simulink library "motohawk_engine_motoshare_lib"  (Simulink 6.3)
undefined symbols (not defined in the file or in its folder): cast_val, IndPowerMax, lookup_group, motohawk_tex, motohawk_vardec_config_group, motohawk_vardec_path, SampleTime, SteadyStateECT, txtTitle, WarmUpTimeConst
libraries: MotoHawk_lib x211, motohawk_control_primitives_lib x20, motohawk_annotations_lib x7, motohawk_engine_lib x5, AutoDoc_lib x4, motohawk_control_primitives_lib_new x3, motohawk_control_primitives_motoshare_lib x2
(part 6 of 7)

== system motohawk_engine_motoshare_lib/Linear Sensor Characterization w Adapt/Faults ==
  RawADC : Inport
  AdaptLimits : Inport  Port=2
  Bus Selector : BusSelector  OutputSignals=adapt_lo_min,adapt_hi_max
  Logical Operator : Logic  AllPortsSameDT=off  OutDataTypeMode=Boolean
  Logical Operator1 : Logic  AllPortsSameDT=off  OutDataTypeMode=Boolean
  Logical Operator2 : Logic  Operator=NOT  AllPortsSameDT=off  OutDataTypeMode=Boolean
  Logical Operator3 : Logic  Operator=NOT  AllPortsSameDT=off  OutDataTypeMode=Boolean
  Relational Operator1 : RelationalOperator  Operator=<
  Relational Operator3 : RelationalOperator  Operator=>
  Relational Operator4 : RelationalOperator  Operator=<
  Relational Operator5 : RelationalOperator  Operator=>
  motohawk_calibration5 : MotoHawk_lib/Calibration & Probing Blocks/motohawk_calibration  nam=[prefix 'RangeHiLimit']  val=1013  storage=Calibration  show_more=on  name_source=Use Parameter  data_type=Inherit from 'Default Value'  read_level=1  write_level=1  ovr_cals=on  view_as=Number  enum_struct={'Disabled', 'Enabled'}  vector_style=Wide Row  use_help_units=on  help='Hi limit of input signal which sets fault'  units='ADC'  use_header_enum=off  row_header_enum={}  col_header_enum={}  use_min_max=off  min_val=-inf  max_val=inf  use_precision=off  precision=''  gain=1  offset=0  exp=1  use_mototune_group=on  mototune_group=[group ' | ' nam ' Config']
  motohawk_calibration6 : MotoHawk_lib/Calibration & Probing Blocks/motohawk_calibration  nam=[prefix 'RangeLoLimit']  val=10  storage=Calibration  show_more=on  name_source=Use Parameter  data_type=Inherit from 'Default Value'  read_level=1  write_level=1  ovr_cals=on  view_as=Number  enum_struct={'Disabled', 'Enabled'}  vector_style=Wide Row  use_help_units=on  help='Low limit of input signal which sets fault'  units='ADC'  use_header_enum=off  row_header_enum={}  col_header_enum={}  use_min_max=off  min_val=-inf  max_val=inf  use_precision=off  precision=''  gain=1  offset=0  exp=1  use_mototune_group=on  mototune_group=[group ' | ' nam ' Config']
  motohawk_fault_def2 : MotoHawk_lib/Fault Management Blocks/motohawk_fault_def  nam=[prefix 'AdaptHi']  mode=Enabled  id=[]  x=25  y=50  input_suspected=on  indeterminate=off  increment_xy=on  downsample_count=1  ovr_cals=on  ovr_actions=on  show_actions=off  action1_name=''  action1_cond=(None)  action2_name=''  action2_cond=(None)  action3_name=''  action3_cond=(None)  action4_name=''  action4_cond=(None)
  motohawk_fault_def4 : MotoHawk_lib/Fault Management Blocks/motohawk_fault_def  nam=[prefix 'RangeHi']  mode=Enabled  id=[]  x=25  y=50  input_suspected=on  indeterminate=off  increment_xy=on  downsample_count=1  ovr_cals=on  ovr_actions=on  show_actions=off  action1_name=''  action1_cond=(None)  action2_name=''  action2_cond=(None)  action3_name=''  action3_cond=(None)  action4_name=''  action4_cond=(None)
  motohawk_fault_def5 : MotoHawk_lib/Fault Management Blocks/motohawk_fault_def  nam=[prefix 'RangeLo']  mode=Enabled  id=[]  x=25  y=50  input_suspected=on  indeterminate=off  increment_xy=on  downsample_count=1  ovr_cals=on  ovr_actions=on  show_actions=off  action1_name=''  action1_cond=(None)  action2_name=''  action2_cond=(None)  action3_name=''  action3_cond=(None)  action4_name=''  action4_cond=(None)
  motohawk_fault_def8 : MotoHawk_lib/Fault Management Blocks/motohawk_fault_def  nam=[prefix 'AdaptLo']  mode=Enabled  id=[]  x=25  y=50  input_suspected=on  indeterminate=off  increment_xy=on  downsample_count=1  ovr_cals=on  ovr_actions=on  show_actions=off  action1_name=''  action1_cond=(None)  action2_name=''  action2_cond=(None)  action3_name=''  action3_cond=(None)  action4_name=''  action4_cond=(None)
  wires:
  AdaptLimits/1 -> Bus Selector/1
  Bus Selector/1 -> Relational Operator1/2  "<adapt_lo_min>"
  Bus Selector/2 -> Relational Operator3/2  "<adapt_hi_max>"
  RawADC/1 -> Relational Operator4/1, Relational Operator5/1, Relational Operator1/1, Relational Operator3/1
  motohawk_calibration6/1 -> Relational Operator4/2
  motohawk_calibration5/1 -> Relational Operator5/2
  Relational Operator4/1 -> motohawk_fault_def5/1, Logical Operator2/1
  Relational Operator5/1 -> motohawk_fault_def4/1, Logical Operator3/1
  Logical Operator/1 -> motohawk_fault_def8/1
  Logical Operator1/1 -> motohawk_fault_def2/1
  Relational Operator1/1 -> Logical Operator/2
  Relational Operator3/1 -> Logical Operator1/2
  Logical Operator2/1 -> Logical Operator/1
  Logical Operator3/1 -> Logical Operator1/1

== system motohawk_engine_motoshare_lib/Load, Torque, Power, Work - Using APC/Calculate Power and Work ==
  IndTorque (N*m) : Inport
  RPM : Inport  Port=2
  Data Type Conversion : DataTypeConversion  SaturateOnIntegerOverflow=on  RndMeth=Zero
  Ground : Ground
  Integrate Power to Compute Work : motohawk_control_primitives_lib/Integrator  samp_time=SampleTime
  Mux1 : Mux  Inputs=2
  Torque to Power : Fcn  Expr=u(1)*u(2)*pi/30000
  motohawk_TitleBlock : motohawk_annotations_lib/motohawk_TitleBlock  BlockType_='Mototron_Title_Block'  ttl='Calculate Observed Engine States, such as Load, Torque, and Power\newline\rmUsing Airflow rate, calculate Air per Cylinder, and lookup Load and Torque values.'  copyright="'THE INFORMATION CONTAINED IN THIS\\newlineDRAWING IS THE SOLE PROPERTY OF\\newlineMOTOTRON.  ANY REPRODUCTION IN\\newline PART OR AS A WHOLE WITHOUT THE\\newlineWRITTEN PERMISSION OF MOTOTRON\\newline IS PROHIBITED.\\fontsize{16}\\rm\\copyright\\rm\\fontsize{10} 2005'"  address='\fontsize{22}\it\fontname{Arial Black}MotoTron Corporation \fontname{Arial}\fontsize{10}\newline505 Marion Road, Oshkosh, WI, 54901\newlinewww.mototron.com (734) 822-7700'  image_file='mh.jpg'  pretty_print=on  edit_text=[motohawk_tex(get_param(bdroot, 'Description')) '\rm\newline' motohawk_tex(get_param(gcs, 'Name'))]  edit_as=6
  motohawk_calibration : MotoHawk_lib/Calibration & Probing Blocks/motohawk_calibration  nam='IndWorkMax'  val=inf  storage=Calibration  show_more=on  name_source=Use Parameter  data_type=Inherit from 'Default Value'  read_level=1  write_level=1  ovr_cals=on  view_as=Number  enum_struct={'Disabled', 'Enabled'}  vector_style=Wide Row  use_help_units=on  help='Maximum Indicated Work'  units='kJ'  use_header_enum=off  row_header_enum={}  col_header_enum={}  use_min_max=off  min_val=-inf  max_val=inf  use_precision=off  precision=''  gain=1  offset=0  exp=1  use_mototune_group=on  mototune_group=lookup_group(gcb)
  motohawk_probe : MotoHawk_lib/Calibration & Probing Blocks/motohawk_probe  nam='IndPower'  show_more=on  name_source=Use Parameter  read_level=1  view_as=Number  enum_struct={'Disabled', 'Enabled'}  vector_style=Wide Row  use_help_units=on  help='Indicated Power'  units='kW'  use_header_enum=off  row_header_enum={}  col_header_enum={}  use_precision=off  precision=''  gain=1  offset=0  exp=1  use_mototune_group=on  mototune_group=lookup_group(gcb)
  motohawk_probe1 : MotoHawk_lib/Calibration & Probing Blocks/motohawk_probe  nam='IndWork'  show_more=on  name_source=Use Parameter  read_level=1  view_as=Number  enum_struct={'Disabled', 'Enabled'}  vector_style=Wide Row  use_help_units=on  help='Indicated Work'  units='kJ'  use_header_enum=off  row_header_enum={}  col_header_enum={}  use_precision=off  precision=''  gain=1  offset=0  exp=1  use_mototune_group=on  mototune_group=lookup_group(gcb)
  IndPower (kW) : Outport
  IndWork (kJ) : Outport  Port=2
  wires:
  Mux1/1 -> Data Type Conversion/1
  Data Type Conversion/1 -> Torque to Power/1
  Torque to Power/1 -> Integrate Power to Compute Work/1, IndPower (kW)/1, motohawk_probe/1
  Integrate Power to Compute Work/1 -> IndWork (kJ)/1, motohawk_probe1/1
  motohawk_calibration/1 -> Integrate Power to Compute Work/5
  IndTorque (N*m)/1 -> Mux1/1
  RPM/1 -> Mux1/2
  Ground/1 -> Integrate Power to Compute Work/3, Integrate Power to Compute Work/2, Integrate Power to Compute Work/4

== system motohawk_engine_motoshare_lib/Mass Flow to Charge Mass Transform/Multiply and Divide, avoiding divde by zero ==
  X1 : Inport
  "X2 " : Inport  Port=2
  Divide1 : Inport  Port=3
  Divide2 : Inport  Port=4
  Enable : EnablePort  StatesWhenEnabling=reset
  charge mass : Product  Inputs=**//  SaturateOnIntegerOverflow=on  InputSameDT=on
  " " : Outport
  wires:
  charge mass/1 -> " "/1
  "X2 "/1 -> charge mass/2
  X1/1 -> charge mass/1
  Divide1/1 -> charge mass/3
  Divide2/1 -> charge mass/4

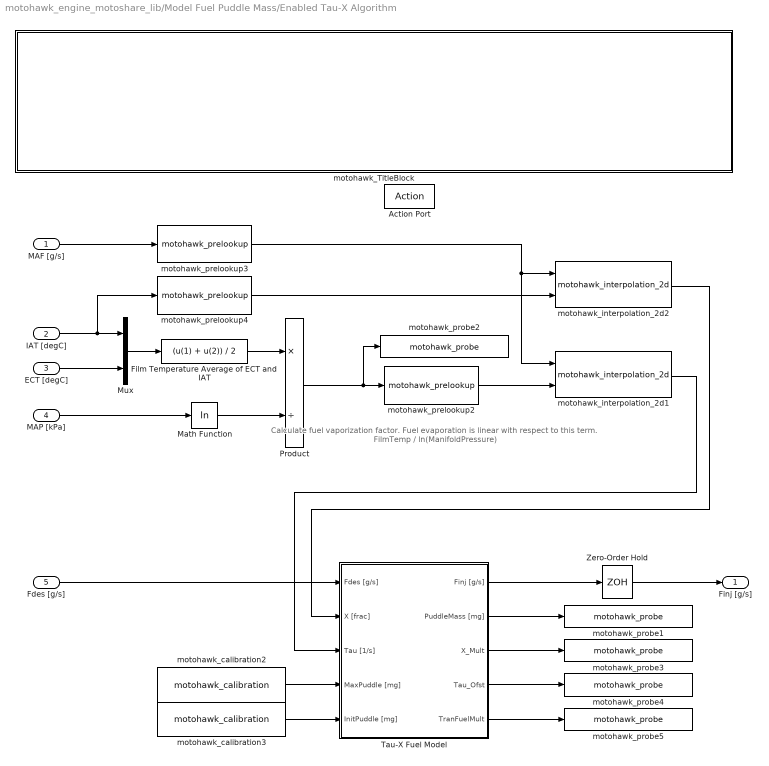
== system motohawk_engine_motoshare_lib/Model Fuel Puddle Mass/Enabled Tau-X Algorithm ==
  note: Calculate fuel vaporization factor.
      | Fuel evaporation is linear with respect to this term.
      | FilmTemp / ln(ManifoldPressure)
  MAF [g/s] : Inport
  IAT [degC] : Inport  Port=2
  ECT [degC] : Inport  Port=3
  MAP [kPa] : Inport  Port=4
  Fdes [g/s] : Inport  Port=5
  Action Port : ActionPort  InitializeStates=reset
  Film Temperature Average of ECT and IAT : Fcn  Expr=(u(1) + u(2)) / 2
  Math Function : Math  Operator=log  SaturateOnIntegerOverflow=on
  Mux : Mux  Inputs=2
  Product : Product  Inputs=*/  SaturateOnIntegerOverflow=on  InputSameDT=on
  Tau-X Fuel Model : Subsystem  mask{samp_time=SampleTime}
      mask prompts: samp_time "Sample Time"
      mask Display:
      | patch([0 0 1 1], 0.5*[0 0.075 0.075 0], [230/255 0/255 0/255])
      | patch([0 0 1 1], 0.5*[0.025 0.05 0.05 0.025], [150/255 0/255 0/255])
      | patch([0 0 1 1], 0.5*[0 0.025 0.025 0], [0/255 0/255 0/255])
      | 
      | disp('TRANSIENT FUELING\nTAU-X MODEL');
  Zero-Order Hold : ZeroOrderHold  SampleTime=-1
  motohawk_TitleBlock : Subsystem  mask{BlockType_='Mototron_Title_Block', ttl=[txtTitle '\newline\rmPer-Cylinder Transient Fueling Model\newlineSchedule Tau and X parameters on RPM and load'], im=mh.jpg}
      mask prompts: ttl "Description"; im "Image FIle"
      mask init:
      | set_param(gcb,'BlockType_','''Mototron_Title_Block''')
      | set_param(gcb,'MaskVisibilityString','off,on,on');
      mask Display:
      | image(imread(im),[0.31 0.66 0.31 0.35])
      | 
      | plot([0 0 1 1 0],[0 1 1 0 0])
      | plot([.3 1],[0.65 0.65])
      | plot([.3 .3],[0.1 1.0])
      | plot([0 1],[0.1 0.1])
      | plot([0.91 0.91],[0 0.1])
      | text(1,1,'\fontsize{22}\it\fontname{Arial Black}MotoTron Corporation \fontname{Arial}\fontsize{10}\newline505 Marion Road, Oshkosh, WI, 54901\newlinewww.mototron.com (734) 822-7700','verticalAlignment','Top','horizontalAlignment','Right','texmode','on')
      | text(0.01,1,['\fontsize{14}\it\bfPROPRIETARY\newlineAND CONFIDENTIAL\newline\fontsize{10}
      | THE INFORMATION CONTAINED IN THIS\newline
      | DRAWING IS THE SOLE PROPERTY OF\newline
      | MOTOTRON.  ANY REPRODUCTION IN\newline
      | PART OR AS A WHOLE WITHOUT THE\newline
      | WRITTEN PERMISSION OF MOTOTRON\newline
      | IS PROHIBITED.\fontsize{16}\rm\copyright\rm\fontsize{10} 2004' ],'verticalAlignment','Top','horizontalAlignment','Left','texmode','on')
      | 
      | text(0.9,0,['\fontsize{11}\bfPath: \rm' strrep(motohawk_vardec_path(gcb),'_','\_')],'verticalAlignment','Bottom','horizontalAlignment','Right','texmode','on')
      | text(0.31,0.65,['\fontsize{10}\bfDescription:'],'verticalAlignment','Top','horizontalAlignment','Left','texmode','on')
      | 
      | text(0.31,0.55,['\fontsize{14}\bf' ttl],'verticalAlignment','Top','horizontalAlignment','Left','texmode','on')
      | text(0.99,0,['\fontsize{11}\bfREV: \rm' motohawk_build_version],'verticalAlignment','Bottom','horizontalAlignment','Right','texmode','on')
  motohawk_calibration2 : MotoHawk_lib/Calibration & Probing Blocks/motohawk_calibration  nam='TransientFuelMaxPuddle'  val=0  storage=Calibration  show_more=on  name_source=Use Parameter  data_type=Inherit from 'Default Value'  read_level=1  write_level=1  ovr_cals=on  view_as=Number  enum_struct={'Disabled', 'Enabled'}  vector_style=Wide Row  use_help_units=on  help='Maximum fuel puddle size'  units='mg'  use_header_enum=off  row_header_enum={}  col_header_enum={}  use_min_max=on  min_val=0  max_val=inf  use_precision=off  precision=''  gain=1  offset=0  exp=1  use_mototune_group=on  mototune_group=group_cal
  motohawk_calibration3 : MotoHawk_lib/Calibration & Probing Blocks/motohawk_calibration  nam='TransientFuelInitPuddle'  val=0  storage=Calibration  show_more=on  name_source=Use Parameter  data_type=Inherit from 'Default Value'  read_level=1  write_level=1  ovr_cals=on  view_as=Number  enum_struct={'Disabled', 'Enabled'}  vector_style=Wide Row  use_help_units=on  help='Initial fuel puddle size'  units='mg'  use_header_enum=off  row_header_enum={}  col_header_enum={}  use_min_max=on  min_val=0  max_val=inf  use_precision=off  precision=''  gain=1  offset=0  exp=1  use_mototune_group=on  mototune_group=group_cal
  motohawk_interpolation_2d1 : MotoHawk_lib/Lookup Tables/motohawk_interpolation_2d  nam='TransientFuelTau'  table_data=ones(5,5)  show_more=on  data_type=Inherit from 'Table Data'  storage=NonAdaptive  read_level=1  write_level=1  ovr_cals=on  use_help=on  help='Fuel evaporation time constant'  units='sec'  use_min_max=on  min_val=SampleTime  max_val=inf  use_precision=off  precision=''  gain=1  offset=0  exp=1  use_links=off  row_prelookup_block=''  col_prelookup_block=''  output_name=''  use_mototune_group=on  mototune_group=group_cal
  motohawk_interpolation_2d2 : MotoHawk_lib/Lookup Tables/motohawk_interpolation_2d  nam='TransientFuelX'  table_data=ones(5,5)  show_more=on  data_type=Inherit from 'Table Data'  storage=NonAdaptive  read_level=1  write_level=1  ovr_cals=on  use_help=on  help='Fraction of injected fuel to enter the puddle'  units='frac'  use_min_max=on  min_val=0  max_val=1  use_precision=off  precision=''  gain=1  offset=0  exp=1  use_links=off  row_prelookup_block=''  col_prelookup_block=''  output_name=''  use_mototune_group=on  mototune_group=group_cal
  motohawk_prelookup2 : MotoHawk_lib/Lookup Tables/motohawk_prelookup  nam='FuelVapFactor'  breakpoint_data=ones(1,5)  show_more=on  data_type=Inherit from 'Table Data'  storage=Constant  read_level=1  write_level=1  ovr_cals=on  use_help=on  help='Breakpoints for fuel vaporization factor'  units='degC/log(kPa)'  use_min_max=off  min_val=-inf  max_val=inf  use_precision=off  precision=''  gain=1  offset=0  exp=1  use_links=on  input_name=''  use_mototune_group=on  mototune_group='Indexes'
  motohawk_prelookup3 : MotoHawk_lib/Lookup Tables/motohawk_prelookup  nam='MAF05'  breakpoint_data=ones(1,5)  show_more=on  data_type=Inherit from 'Table Data'  storage=Constant  read_level=1  write_level=1  ovr_cals=on  use_help=on  help='Breakpoints for Mass Airflow'  units='g/s'  use_min_max=off  min_val=-inf  max_val=inf  use_precision=off  precision=''  gain=1  offset=0  exp=1  use_links=on  input_name='MAF'  use_mototune_group=on  mototune_group='Indexes'
  motohawk_prelookup4 : MotoHawk_lib/Lookup Tables/motohawk_prelookup  nam='IAT05'  breakpoint_data=ones(1,5)  show_more=on  data_type=Inherit from 'Table Data'  storage=Constant  read_level=1  write_level=1  ovr_cals=on  use_help=on  help='Breakpoints for intake air temperature'  units='degC'  use_min_max=off  min_val=-inf  max_val=inf  use_precision=off  precision=''  gain=1  offset=0  exp=1  use_links=on  input_name='IAT'  use_mototune_group=on  mototune_group='Indexes'
  motohawk_probe1 : MotoHawk_lib/Calibration & Probing Blocks/motohawk_probe  nam='TransientFuelPuddleMass'  show_more=on  name_source=Use Parameter  read_level=1  view_as=Number  enum_struct={'Disabled', 'Enabled'}  vector_style=Wide Row  use_help_units=on  help='Current modeled fuel puddle mass for Tau-X transient fuel'  units='mg'  use_header_enum=off  row_header_enum={}  col_header_enum={}  use_precision=off  precision=''  gain=1  offset=0  exp=1  use_mototune_group=on  mototune_group=group_dis
  motohawk_probe2 : MotoHawk_lib/Calibration & Probing Blocks/motohawk_probe  nam='FuelVapFactor'  show_more=on  name_source=Use Parameter  read_level=1  view_as=Number  enum_struct={'Disabled', 'Enabled'}  vector_style=Wide Row  use_help_units=on  help='Fuel vaporization factor - Fuel evaporation is linear with respect to this term'  units='degC/log(kPa)'  use_header_enum=off  row_header_enum={}  col_header_enum={}  use_precision=off  precision=''  gain=1  offset=0  exp=1  use_mototune_group=on  mototune_group=group_dis
  motohawk_probe3 : MotoHawk_lib/Calibration & Probing Blocks/motohawk_probe  nam='TransientFuel_X_Mult'  show_more=on  name_source=Use Parameter  read_level=1  view_as=Number  enum_struct={'Disabled', 'Enabled'}  vector_style=Wide Row  use_help_units=on  help='Multiplier on desired fuel flow due to X contribution (1/(1-X)).'  units=''  use_header_enum=off  row_header_enum={}  col_header_enum={}  use_precision=off  precision=''  gain=1  offset=0  exp=1  use_mototune_group=on  mototune_group=group_dis
  motohawk_probe4 : MotoHawk_lib/Calibration & Probing Blocks/motohawk_probe  nam='TransientFuel_Tau_Ofst'  show_more=on  name_source=Use Parameter  read_level=1  view_as=Number  enum_struct={'Disabled', 'Enabled'}  vector_style=Wide Row  use_help_units=on  help='Offset applied to desired fuel flow based on Tau contribution (-M_pud/Tau).'  units='g/s'  use_header_enum=off  row_header_enum={}  col_header_enum={}  use_precision=off  precision=''  gain=1  offset=0  exp=1  use_mototune_group=on  mototune_group=group_dis
  motohawk_probe5 : MotoHawk_lib/Calibration & Probing Blocks/motohawk_probe  nam='TransientFuel_Total_Mult'  show_more=on  name_source=Use Parameter  read_level=1  view_as=Number  enum_struct={'Disabled', 'Enabled'}  vector_style=Wide Row  use_help_units=on  help='Total transient fuel multiplier applied to desired fuel flow resulting from Tau-X model.'  units=''  use_header_enum=off  row_header_enum={}  col_header_enum={}  use_precision=off  precision=''  gain=1  offset=0  exp=1  use_mototune_group=on  mototune_group=group_dis
  Finj [g/s] : Outport
  wires:
  Tau-X Fuel Model/5(TranFuelMult) -> motohawk_probe5/1
  Tau-X Fuel Model/4(Tau_Ofst) -> motohawk_probe4/1
  Tau-X Fuel Model/3(X_Mult) -> motohawk_probe3/1
  motohawk_calibration2/1 -> Tau-X Fuel Model/4(MaxPuddle [mg])
  motohawk_calibration3/1 -> Tau-X Fuel Model/5(InitPuddle [mg])
  Tau-X Fuel Model/2(PuddleMass [mg]) -> motohawk_probe1/1
  Mux/1 -> Film Temperature Average of ECT and IAT/1
  Film Temperature Average of ECT and IAT/1 -> Product/1
  Math Function/1 -> Product/2
  Product/1 -> motohawk_prelookup2/1, motohawk_probe2/1
  IAT [degC]/1 -> Mux/1, motohawk_prelookup4/1
  motohawk_prelookup3/1 -> motohawk_interpolation_2d2/1, motohawk_interpolation_2d1/1
  motohawk_prelookup4/1 -> motohawk_interpolation_2d2/2
  Fdes [g/s]/1 -> Tau-X Fuel Model/1(Fdes [g/s])
  MAF [g/s]/1 -> motohawk_prelookup3/1
  ECT [degC]/1 -> Mux/2
  MAP [kPa]/1 -> Math Function/1
  Tau-X Fuel Model/1(Finj [g/s]) -> Zero-Order Hold/1
  Zero-Order Hold/1 -> Finj [g/s]/1
  motohawk_prelookup2/1 -> motohawk_interpolation_2d1/2
  motohawk_interpolation_2d1/1 -> Tau-X Fuel Model/3(Tau [1/s])
  motohawk_interpolation_2d2/1 -> Tau-X Fuel Model/2(X [frac])

== system motohawk_engine_motoshare_lib/Model Fuel Puddle Mass/Pass-Through ==
  note: Simply pass-through desired fuel as injected fuel
      | when transient fueling is disabled
  Fdes [g/s] : Inport
  Action Port : ActionPort  InitializeStates=reset
  Finj [g/s] : Outport
  wires:
  Fdes [g/s]/1 -> Finj [g/s]/1

== system motohawk_engine_motoshare_lib/Model Fuel Puddle Mass/motohawk_TitleBlock ==

== system motohawk_engine_motoshare_lib/Non-Linear Sensor Characterization (eqn)/If Action Subsystem ==
  In : Inport
  Action Port : ActionPort
  Out : Outport
  wires:
  In/1 -> Out/1

== system motohawk_engine_motoshare_lib/Non-Linear Sensor Characterization (eqn)/If Action Subsystem2 ==
  In : Inport
  Action Port : ActionPort
  Out : Outport
  wires:
  In/1 -> Out/1

== system motohawk_engine_motoshare_lib/Non-Linear Sensor Characterization (tbl)/If Action Subsystem ==
  In : Inport
  Action Port : ActionPort
  Out : Outport
  wires:
  In/1 -> Out/1

== system motohawk_engine_motoshare_lib/Non-Linear Sensor Characterization (tbl)/If Action Subsystem1 ==
  In : Inport
  Action Port : ActionPort
  Out : Outport
  wires:
  In/1 -> Out/1

== system motohawk_engine_motoshare_lib/Non-Linear Sensor Characterization (tbl)/If Action Subsystem2 ==
  In : Inport
  Action Port : ActionPort
  Out : Outport
  wires:
  In/1 -> Out/1

== system motohawk_engine_motoshare_lib/Normalized Effective Combustion Chamber Temperature/CompareTo ==
  note: Check how input compares to 'val'
  In : Inport
  Constant : Constant  Value=val
  RelOp : RelationalOperator  Operator===  ZeroCross=off  InputSameDT=on
  Out : Outport
  wires:
  In/1 -> RelOp/1
  RelOp/1 -> Out/1
  Constant/1 -> RelOp/2

== system motohawk_engine_motoshare_lib/Normalized Effective Combustion Chamber Temperature/Integrate an offset to ECT  Reset offset when engine is stopped. ==
  Integrand : Inport
  Reset : Inport  Port=2
  Enable : EnablePort
  Constant : Constant  Value=0
  Constant1 : Constant  Value=0
  Constant2 : Constant  Value=inf
  Integrator : Subsystem  mask(Discrete Integrator){samp_time=SampleTime}
      mask prompts: samp_time "Sample Time"
      mask help:
      | Resetable integrator with upper and lower windup limits.
      |
      | If 'Sample Time' is -1, then extra code and RAM will be generated to dynamically calculate dt.
      mask Display:
      | patch([0 0 1 1], 0.75*[0 0.075 0.075 0], [230/255 0/255 0/255])
      | patch([0 0 1 1], 0.75*[0.025 0.05 0.05 0.025], [150/255 0/255 0/255])
      | patch([0 0 1 1], 0.75*[0 0.025 0.025 0], [0/255 0/255 0/255])
      | 
      | disp('\fontsize{16}\bf\it\int dt', 'texmode', 'on')
  ECT Offset : Outport
  wires:
  Constant/1 -> Integrator/4(Min)
  Constant1/1 -> Integrator/3(IC)
  Integrand/1 -> Integrator/1(In)
  Integrator/1(Out) -> ECT Offset/1
  Reset/1 -> Integrator/2(Rst)
  Constant2/1 -> Integrator/5(Max)

== system motohawk_engine_motoshare_lib/Normalized Effective Combustion Chamber Temperature/motohawk_TitleBlock ==

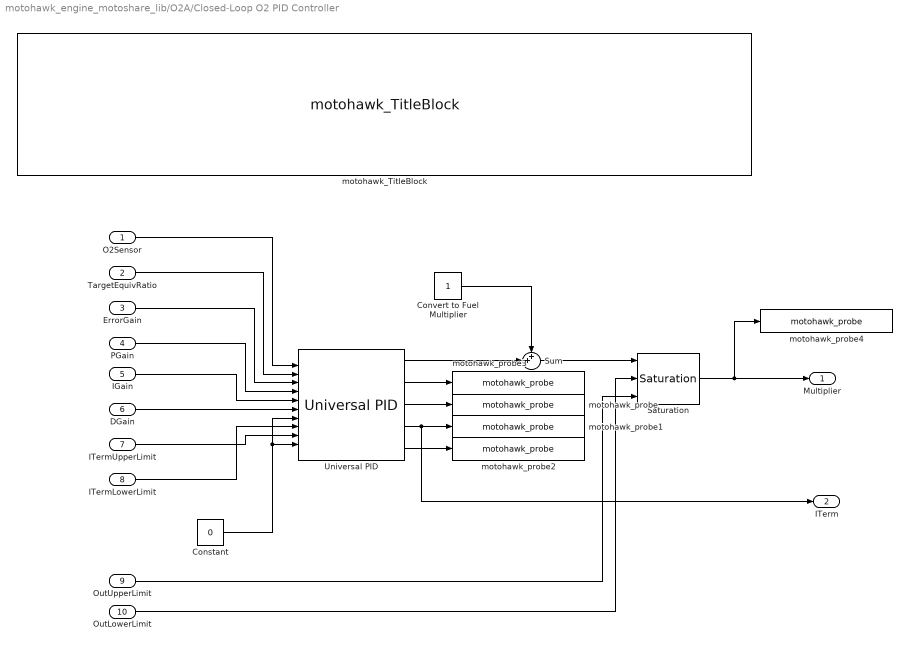
== system motohawk_engine_motoshare_lib/O2A/Closed-Loop O2 PID Controller ==
  O2Sensor : Inport
  TargetEquivRatio : Inport  Port=2
  ErrorGain : Inport  Port=3
  PGain : Inport  Port=4
  IGain : Inport  Port=5
  DGain : Inport  Port=6
  ITermUpperLimit : Inport  Port=7
  ITermLowerLimit : Inport  Port=8
  OutUpperLimit : Inport  Port=9
  OutLowerLimit : Inport  Port=10
  Constant : Constant  Value=0
  Convert to Fuel Multiplier : Constant
  Saturation : motohawk_control_primitives_lib/Saturation
  Sum : Sum  Inputs=++|  SaturateOnIntegerOverflow=on  InputSameDT=on
  Universal PID : motohawk_control_primitives_lib/Universal PID  Description=|  samp_time=-1
      | /* Name: ErrorGain Unit:mult ClassID:VAR StorageID:FLASH Access:RW4+RW3+NA2+NA1 TypeID:UINT4                   
      |    Gain:0.000000001 Min:0.000000000 Max:4.000000000 Format:10.9 UpdateID:REMOTE Help:"This gain is applied to "
      |    "the error term before it is used to calculate the P, I and D terms." VardecSig:6C */                       
      |                                                                                                                
      | /* Name: ITermLowerLim Unit:0 ClassID:VAR StorageID:FLASH Access:RW4+RW3+NA2+NA1 TypeID:SINT2 Gain:0.1         
      |    Min:-3276.8 Max:3276.7 Format:5.1 UpdateID:REMOTE Help:"Lower limit on the I-term value." VardecSig:6C */   
      |                                                                                                                
      | /* Name: ITermUpperLim ClassID:VAR StorageID:FLASH Access:RW4+RW3+NA2+NA1 TypeID:SINT2 Gain:0.1 Min:-3276.8    
      |    Max:3276.7 Format:5.1 UpdateID:REMOTE Help:"Upper limit on I-term value." VardecSig:6C */                   
      |                                                                                                                
      | /* Name: PIDOutLowerLim ClassID:VAR StorageID:FLASH Access:RW4+RW3+NA2+NA1 TypeID:SINT2 Gain:0.1               
      |    Min:-3276.8 Max:3276.7 Format:5.1 UpdateID:REMOTE Help:"Lower limit on PID output." VardecSig:6C */         
      |                                                                                                                
      | /* Name: PIDOutUpperLim ClassID:VAR StorageID:FLASH Access:RW4+RW3+NA2+NA1 TypeID:SINT2 Gain:0.1               
      |    Min:-3276.8 Max:3276.7 Format:3.1 UpdateID:REMOTE Help:"Upper limit on PID output." VardecSig:6C */
  motohawk_TitleBlock : motohawk_annotations_lib/motohawk_TitleBlock  BlockType_='Mototron_Title_Block'  ttl=[txtTitle '\newline\rmClosed-loop O2 Control - PID for Bank A']  copyright="'THE INFORMATION CONTAINED IN THIS\\newlineDRAWING IS THE SOLE PROPERTY OF\\newlineMOTOTRON.  ANY REPRODUCTION IN\\newline PART OR AS A WHOLE WITHOUT THE\\newlineWRITTEN PERMISSION OF MOTOTRON\\newline IS PROHIBITED.\\fontsize{16}\\rm\\copyright\\rm\\fontsize{10} 2005'"  address='\fontsize{22}\it\fontname{Arial Black}MotoTron Corporation \fontname{Arial}\fontsize{10}\newline505 Marion Road, Oshkosh, WI, 54901\newlinewww.mototron.com (734) 822-7700'  image_file='mh.jpg'  pretty_print=on  edit_text=[motohawk_tex(get_param(bdroot, 'Description')) '\rm\newline' motohawk_tex(get_param(gcs, 'Name'))]  edit_as=6
  motohawk_probe : MotoHawk_lib/Calibration & Probing Blocks/motohawk_probe  nam=['O2Control_PTerm' bank]  show_more=on  name_source=Use Parameter  read_level=1  view_as=Number  enum_struct={'Disabled', 'Enabled'}  vector_style=Wide Row  use_help_units=on  help=['Closed-loop O2 control P-Term, for bank ' bank]  units='mult'  use_header_enum=off  row_header_enum={}  col_header_enum={}  use_precision=off  precision=''  gain=1  offset=0  exp=1  use_mototune_group=on  mototune_group=display_group
  motohawk_probe1 : MotoHawk_lib/Calibration & Probing Blocks/motohawk_probe  nam=['O2Control_ITerm' bank]  show_more=on  name_source=Use Parameter  read_level=1  view_as=Number  enum_struct={'Disabled', 'Enabled'}  vector_style=Wide Row  use_help_units=on  help=['Closed-loop O2 control I-Term, for bank ' bank]  units='mult'  use_header_enum=off  row_header_enum={}  col_header_enum={}  use_precision=off  precision=''  gain=1  offset=0  exp=1  use_mototune_group=on  mototune_group=display_group
  motohawk_probe2 : MotoHawk_lib/Calibration & Probing Blocks/motohawk_probe  nam=['O2Control_DTerm' bank]  show_more=on  name_source=Use Parameter  read_level=1  view_as=Number  enum_struct={'Disabled', 'Enabled'}  vector_style=Wide Row  use_help_units=on  help=['Closed-loop O2 control D-Term, for bank ' bank]  units='mult'  use_header_enum=off  row_header_enum={}  col_header_enum={}  use_precision=off  precision=''  gain=1  offset=0  exp=1  use_mototune_group=on  mototune_group=display_group
  motohawk_probe3 : MotoHawk_lib/Calibration & Probing Blocks/motohawk_probe  nam=['O2Control_ErrorTerm' bank]  show_more=on  name_source=Use Parameter  read_level=1  view_as=Number  enum_struct={'Disabled', 'Enabled'}  vector_style=Wide Row  use_help_units=on  help=['Closed-loop O2 control error-term, for bank ' bank]  units='mult'  use_header_enum=off  row_header_enum={}  col_header_enum={}  use_precision=off  precision=''  gain=1  offset=0  exp=1  use_mototune_group=on  mototune_group=display_group
  motohawk_probe4 : MotoHawk_lib/Calibration & Probing Blocks/motohawk_probe  nam=['O2FuelMult' bank]  show_more=on  name_source=Use Parameter  read_level=1  view_as=Number  enum_struct={'Disabled', 'Enabled'}  vector_style=Wide Row  use_help_units=on  help=['Closed-loop O2 control fuel multiplier, for bank ' bank]  units='mult'  use_header_enum=off  row_header_enum={}  col_header_enum={}  use_precision=off  precision=''  gain=1  offset=0  exp=1  use_mototune_group=on  mototune_group=display_group
  Multiplier : Outport
  ITerm : Outport  Port=2
  wires:
  Universal PID/2 -> motohawk_probe3/1
  OutLowerLimit/1 -> Saturation/2
  ITermLowerLimit/1 -> Universal PID/8
  ITermUpperLimit/1 -> Universal PID/9
  Sum/1 -> Saturation/1
  Universal PID/1 -> Sum/2
  Convert to Fuel Multiplier/1 -> Sum/1
  OutUpperLimit/1 -> Saturation/3
  DGain/1 -> Universal PID/6
  IGain/1 -> Universal PID/5
  PGain/1 -> Universal PID/4
  ErrorGain/1 -> Universal PID/3
  TargetEquivRatio/1 -> Universal PID/2
  O2Sensor/1 -> Universal PID/1
  Saturation/1 -> motohawk_probe4/1, Multiplier/1
  Universal PID/5 -> motohawk_probe2/1
  Constant/1 -> Universal PID/7, Universal PID/10
  Universal PID/4 -> ITerm/1, motohawk_probe1/1
  Universal PID/3 -> motohawk_probe/1

== system motohawk_engine_motoshare_lib/O2A/Equivalence Ratio Perturbation ==
  note: When low, switch to rich.
      | When high, switch to lean.
  O2Sensor : Inport
  DesEquivRatio : Inport  Port=2
  RichEquivRatioTargetDelta : Inport  Port=3
  LeanEquivRatioTargetDelta : Inport  Port=4
  RichEquivRatioSwPtDelta : Inport  Port=5
  LeanEquivRatioSwPtDelta : Inport  Port=6
  Hysteresis : Subsystem
  LT : RelationalOperator  ZeroCross=off  InputSameDT=on
  LT1 : RelationalOperator  Operator=<=  ZeroCross=off  InputSameDT=on
  Logical Operator : Logic  Operator=NOT
  Sum1 : Sum  SaturateOnIntegerOverflow=on
  Sum2 : Sum  Inputs=-+  SaturateOnIntegerOverflow=on
  Sum3 : Sum  SaturateOnIntegerOverflow=on
  Sum4 : Sum  Inputs=+-  SaturateOnIntegerOverflow=on
  Switch2 : Switch  Threshold=1  ZeroCross=off  InputSameDT=on
  motohawk_TitleBlock : motohawk_annotations_lib/motohawk_TitleBlock  BlockType_='Mototron_Title_Block'  ttl=[txtTitle '\newline\rmO2 Control Target Equivalence Ratio Perturbation around Stoichiometric']  copyright="'THE INFORMATION CONTAINED IN THIS\\newlineDRAWING IS THE SOLE PROPERTY OF\\newlineMOTOTRON.  ANY REPRODUCTION IN\\newline PART OR AS A WHOLE WITHOUT THE\\newlineWRITTEN PERMISSION OF MOTOTRON\\newline IS PROHIBITED.\\fontsize{16}\\rm\\copyright\\rm\\fontsize{10} 2005'"  address='\fontsize{22}\it\fontname{Arial Black}MotoTron Corporation \fontname{Arial}\fontsize{10}\newline505 Marion Road, Oshkosh, WI, 54901\newlinewww.mototron.com (734) 822-7700'  image_file='mh.jpg'  pretty_print=on  edit_text=[motohawk_tex(get_param(bdroot, 'Description')) '\rm\newline' motohawk_tex(get_param(gcs, 'Name'))]  edit_as=6
  motohawk_fault_def : MotoHawk_lib/Fault Management Blocks/motohawk_fault_def  nam=['O2FailedLean',bank]  mode=Enabled  id=[]  x=25  y=50  input_suspected=on  indeterminate=off  increment_xy=on  downsample_count=1  ovr_cals=on  ovr_actions=on  show_actions=off  action1_name=''  action1_cond=(None)  action2_name=''  action2_cond=(None)  action3_name=''  action3_cond=(None)  action4_name=''  action4_cond=(None)
  motohawk_fault_def1 : MotoHawk_lib/Fault Management Blocks/motohawk_fault_def  nam=['O2FailedRich',bank]  mode=Enabled  id=[]  x=25  y=50  input_suspected=on  indeterminate=off  increment_xy=on  downsample_count=1  ovr_cals=on  ovr_actions=on  show_actions=off  action1_name=''  action1_cond=(None)  action2_name=''  action2_cond=(None)  action3_name=''  action3_cond=(None)  action4_name=''  action4_cond=(None)
  Target Phi : Outport
  wires:
  Logical Operator/1 -> Switch2/2
  O2Sensor/1 -> LT/1, LT1/1
  Hysteresis/1("Out (Lo=0, Hi=1)") -> Logical Operator/1
  LT1/1 -> motohawk_fault_def/1, Hysteresis/2(Lo)  "BelowLean"
  LT/1 -> motohawk_fault_def1/1, Hysteresis/1(Hi)  "AboveRich"
  RichEquivRatioTargetDelta/1 -> Sum1/1
  LeanEquivRatioTargetDelta/1 -> Sum2/1
  Sum1/1 -> Switch2/1
  Sum2/1 -> Switch2/3
  LeanEquivRatioSwPtDelta/1 -> Sum4/2
  RichEquivRatioSwPtDelta/1 -> Sum3/2
  DesEquivRatio/1 -> Sum3/1, Sum4/1, Sum2/2, Sum1/2
  Switch2/1 -> Target Phi/1
  Sum4/1 -> LT1/2
  Sum3/1 -> LT/2

== system motohawk_engine_motoshare_lib/O2A/O2 Calibrations ==
  Bus Creator : BusCreator  Inputs=12
  motohawk_TitleBlock : motohawk_annotations_lib/motohawk_TitleBlock  BlockType_='Mototron_Title_Block'  ttl=[txtTitle '\newline\rmClosed-Loop O2 Control Calibrations']  copyright="'THE INFORMATION CONTAINED IN THIS\\newlineDRAWING IS THE SOLE PROPERTY OF\\newlineMOTOTRON.  ANY REPRODUCTION IN\\newline PART OR AS A WHOLE WITHOUT THE\\newlineWRITTEN PERMISSION OF MOTOTRON\\newline IS PROHIBITED.\\fontsize{16}\\rm\\copyright\\rm\\fontsize{10} 2005'"  address='\fontsize{22}\it\fontname{Arial Black}MotoTron Corporation \fontname{Arial}\fontsize{10}\newline505 Marion Road, Oshkosh, WI, 54901\newlinewww.mototron.com (734) 822-7700'  image_file='mh.jpg'  pretty_print=on  edit_text=[motohawk_tex(get_param(bdroot, 'Description')) '\rm\newline' motohawk_tex(get_param(gcs, 'Name'))]  edit_as=6
  motohawk_calibration1 : MotoHawk_lib/Calibration & Probing Blocks/motohawk_calibration  nam=['LeanEquivRatioTargetDelta' bank]  val=.05  storage=Calibration  show_more=on  name_source=Use Parameter  data_type=Inherit from 'Default Value'  read_level=1  write_level=1  ovr_cals=on  view_as=Number  enum_struct={'Disabled', 'Enabled'}  vector_style=Wide Row  use_help_units=on  help='Target equivalence ratio below desired, when driving lean'  units='ratio'  use_header_enum=off  row_header_enum={}  col_header_enum={}  use_min_max=on  min_val=0  max_val=1.0  use_precision=off  precision=''  gain=1  offset=0  exp=1  use_mototune_group=on  mototune_group=cal_group
  motohawk_calibration10 : MotoHawk_lib/Calibration & Probing Blocks/motohawk_calibration  nam=['O2ControlOutUpperLimit',bank]  val=1.4  storage=Calibration  show_more=on  name_source=Use Parameter  data_type=Inherit from 'Default Value'  read_level=1  write_level=1  ovr_cals=on  view_as=Number  enum_struct={'Disabled', 'Enabled'}  vector_style=Wide Row  use_help_units=on  help='PID fuel multiplier output upper limit for closed-loop O2 control'  units='mult'  use_header_enum=off  row_header_enum={}  col_header_enum={}  use_min_max=on  min_val=-inf  max_val=inf  use_precision=off  precision=''  gain=1  offset=0  exp=1  use_mototune_group=on  mototune_group=cal_group
  motohawk_calibration11 : MotoHawk_lib/Calibration & Probing Blocks/motohawk_calibration  nam=['O2ControlOutLowerLimit',bank]  val=.6  storage=Calibration  show_more=on  name_source=Use Parameter  data_type=Inherit from 'Default Value'  read_level=1  write_level=1  ovr_cals=on  view_as=Number  enum_struct={'Disabled', 'Enabled'}  vector_style=Wide Row  use_help_units=on  help='PID fuel multiplier output lower limit for closed-loop O2 control'  units='mult'  use_header_enum=off  row_header_enum={}  col_header_enum={}  use_min_max=on  min_val=-inf  max_val=inf  use_precision=off  precision=''  gain=1  offset=0  exp=1  use_mototune_group=on  mototune_group=cal_group
  motohawk_calibration12 : MotoHawk_lib/Calibration & Probing Blocks/motohawk_calibration  nam=['RichEquivRatioTargetDelta' bank]  val=.05  storage=Calibration  show_more=on  name_source=Use Parameter  data_type=Inherit from 'Default Value'  read_level=1  write_level=1  ovr_cals=on  view_as=Number  enum_struct={'Disabled', 'Enabled'}  vector_style=Wide Row  use_help_units=on  help='Target equivalence ratio below desired, when driving lean'  units='ratio'  use_header_enum=off  row_header_enum={}  col_header_enum={}  use_min_max=on  min_val=0  max_val=1.0  use_precision=off  precision=''  gain=1  offset=0  exp=1  use_mototune_group=on  mototune_group=cal_group
  motohawk_calibration2 : MotoHawk_lib/Calibration & Probing Blocks/motohawk_calibration  nam=['RichEquivRatioSwPtDelta',bank]  val=.01  storage=Calibration  show_more=on  name_source=Use Parameter  data_type=Inherit from 'Default Value'  read_level=1  write_level=1  ovr_cals=on  view_as=Number  enum_struct={'Disabled', 'Enabled'}  vector_style=Wide Row  use_help_units=on  help='Switch point equivalence ratio above desired, when driving rich, and changing to lean'  units='ratio'  use_header_enum=off  row_header_enum={}  col_header_enum={}  use_min_max=on  min_val=0  max_val=1.0  use_precision=off  precision=''  gain=1  offset=0  exp=1  use_mototune_group=on  mototune_group=cal_group
  motohawk_calibration3 : MotoHawk_lib/Calibration & Probing Blocks/motohawk_calibration  nam=['LeanEquivRatioSwPtDelta',bank]  val=.01  storage=Calibration  show_more=on  name_source=Use Parameter  data_type=Inherit from 'Default Value'  read_level=1  write_level=1  ovr_cals=on  view_as=Number  enum_struct={'Disabled', 'Enabled'}  vector_style=Wide Row  use_help_units=on  help='Switch point equivalence ratio below desired, when driving lean, and changing to rich'  units='ratio'  use_header_enum=off  row_header_enum={}  col_header_enum={}  use_min_max=on  min_val=0  max_val=1.0  use_precision=off  precision=''  gain=1  offset=0  exp=1  use_mototune_group=on  mototune_group=cal_group
  motohawk_calibration4 : MotoHawk_lib/Calibration & Probing Blocks/motohawk_calibration  nam=['O2ControlErrorGain',bank]  val=.2  storage=Calibration  show_more=on  name_source=Use Parameter  data_type=Inherit from 'Default Value'  read_level=1  write_level=1  ovr_cals=on  view_as=Number  enum_struct={'Disabled', 'Enabled'}  vector_style=Wide Row  use_help_units=on  help='PID error gain for closed-loop O2 control'  units='mult'  use_header_enum=off  row_header_enum={}  col_header_enum={}  use_min_max=on  min_val=-inf  max_val=inf  use_precision=off  precision=''  gain=1  offset=0  exp=1  use_mototune_group=on  mototune_group=cal_group
  motohawk_calibration5 : MotoHawk_lib/Calibration & Probing Blocks/motohawk_calibration  nam=['O2ControlPGain',bank]  val=1  storage=Calibration  show_more=on  name_source=Use Parameter  data_type=Inherit from 'Default Value'  read_level=1  write_level=1  ovr_cals=on  view_as=Number  enum_struct={'Disabled', 'Enabled'}  vector_style=Wide Row  use_help_units=on  help='PID P-Term gain for closed-loop O2 control'  units='mult'  use_header_enum=off  row_header_enum={}  col_header_enum={}  use_min_max=on  min_val=-inf  max_val=inf  use_precision=off  precision=''  gain=1  offset=0  exp=1  use_mototune_group=on  mototune_group=cal_group
  motohawk_calibration6 : MotoHawk_lib/Calibration & Probing Blocks/motohawk_calibration  nam=['O2ControlIGain',bank]  val=2  storage=Calibration  show_more=on  name_source=Use Parameter  data_type=Inherit from 'Default Value'  read_level=1  write_level=1  ovr_cals=on  view_as=Number  enum_struct={'Disabled', 'Enabled'}  vector_style=Wide Row  use_help_units=on  help='PID I-Term gain for closed-loop O2 control'  units='mult'  use_header_enum=off  row_header_enum={}  col_header_enum={}  use_min_max=on  min_val=-inf  max_val=inf  use_precision=off  precision=''  gain=1  offset=0  exp=1  use_mototune_group=on  mototune_group=cal_group
  motohawk_calibration7 : MotoHawk_lib/Calibration & Probing Blocks/motohawk_calibration  nam=['O2ControlDGain',bank]  val=0  storage=Calibration  show_more=on  name_source=Use Parameter  data_type=Inherit from 'Default Value'  read_level=1  write_level=1  ovr_cals=on  view_as=Number  enum_struct={'Disabled', 'Enabled'}  vector_style=Wide Row  use_help_units=on  help='PID D-Term gain for closed-loop O2 control'  units='mult'  use_header_enum=off  row_header_enum={}  col_header_enum={}  use_min_max=on  min_val=-inf  max_val=inf  use_precision=off  precision=''  gain=1  offset=0  exp=1  use_mototune_group=on  mototune_group=cal_group
  motohawk_calibration8 : MotoHawk_lib/Calibration & Probing Blocks/motohawk_calibration  nam=['O2ControlITermLowerLimit',bank]  val=-.4  storage=Calibration  show_more=on  name_source=Use Parameter  data_type=Inherit from 'Default Value'  read_level=1  write_level=1  ovr_cals=on  view_as=Number  enum_struct={'Disabled', 'Enabled'}  vector_style=Wide Row  use_help_units=on  help='PID I-Term lower limit for closed-loop O2 control'  units='mult'  use_header_enum=off  row_header_enum={}  col_header_enum={}  use_min_max=on  min_val=-inf  max_val=inf  use_precision=off  precision=''  gain=1  offset=0  exp=1  use_mototune_group=on  mototune_group=cal_group
  motohawk_calibration9 : MotoHawk_lib/Calibration & Probing Blocks/motohawk_calibration  nam=['O2ControlITermUpperLimit',bank]  val=.3  storage=Calibration  show_more=on  name_source=Use Parameter  data_type=Inherit from 'Default Value'  read_level=1  write_level=1  ovr_cals=on  view_as=Number  enum_struct={'Disabled', 'Enabled'}  vector_style=Wide Row  use_help_units=on  help='PID I-Term upper limit for closed-loop O2 control'  units='mult'  use_header_enum=off  row_header_enum={}  col_header_enum={}  use_min_max=on  min_val=-inf  max_val=inf  use_precision=off  precision=''  gain=1  offset=0  exp=1  use_mototune_group=on  mototune_group=cal_group
  Calibrations : Outport
  wires:
  motohawk_calibration12/1 -> Bus Creator/1  "RichEquivRatioTargetDelta"
  Bus Creator/1 -> Calibrations/1
  motohawk_calibration11/1 -> Bus Creator/12  "O2ControlOutLowerLimit"
  motohawk_calibration10/1 -> Bus Creator/11  "O2ControlOutUpperLimit"
  motohawk_calibration8/1 -> Bus Creator/10  "O2ControlItermLowerLimit"
  motohawk_calibration9/1 -> Bus Creator/9  "O2ControlITermUpperLimit"
  motohawk_calibration7/1 -> Bus Creator/8  "O2ControlDGain"
  motohawk_calibration6/1 -> Bus Creator/7  "O2ControlIGain"
  motohawk_calibration5/1 -> Bus Creator/6  "O2ControlPGain"
  motohawk_calibration4/1 -> Bus Creator/5  "O2ControlErrorGain"
  motohawk_calibration3/1 -> Bus Creator/4  "LeanEquivRatioSwPtDelta"
  motohawk_calibration2/1 -> Bus Creator/3  "RichEquivRatioSwPtDelta"
  motohawk_calibration1/1 -> Bus Creator/2  "LeanEquivRatioTargetDelta"

== system motohawk_engine_motoshare_lib/Speed Density - MAP Referenced - Adaptive/Adapt Volumetric Efficiency ==
  SSEngOpr [bool] : Inport
  MAF_Sensor [g/s] : Inport  Port=2
  MAF_Model [g/s] : Inport  Port=3
  VE : Inport  Port=4
  Abs : Abs  SaturateOnIntegerOverflow=on
  Adapt VolEff Map : Subsystem
  Logical Operator : Logic  Inputs=3
  Product0 : Product  SaturateOnIntegerOverflow=on  InputSameDT=on
  Relational Operator : RelationalOperator  Operator=<=  InputSameDT=on
  Safe Divide : Subsystem
  Sum1 : Sum  Inputs=+-  SaturateOnIntegerOverflow=on  InputSameDT=on
  motohawk_calibration : MotoHawk_lib/Calibration & Probing Blocks/motohawk_calibration  nam='VEAdaptEnable'  val=false  storage=Display  show_more=on  name_source=Use Parameter  data_type=Inherit from 'Default Value'  read_level=1  write_level=1  ovr_cals=on  view_as=Enumeration  enum_struct={'Disabled', 'Enabled'}  vector_style=Wide Row  use_help_units=on  help='Determines whether the Volumetric Efficiency map will be adapted using the MAF sensor'  units='bool'  use_header_enum=off  row_header_enum={}  col_header_enum={}  use_min_max=off  min_val=-inf  max_val=inf  use_precision=off  precision=''  gain=1  offset=0  exp=1  use_mototune_group=on  mototune_group=lookup_group(gcb)
  motohawk_calibration1 : MotoHawk_lib/Calibration & Probing Blocks/motohawk_calibration  nam='VEAdaptDelta'  val=1  storage=Calibration  show_more=on  name_source=Use Parameter  data_type=Inherit from 'Default Value'  read_level=1  write_level=1  ovr_cals=on  view_as=Number  enum_struct={'Disabled', 'Enabled'}  vector_style=Wide Row  use_help_units=on  help='VolEff_Error must be less than this delta to adapt the VolEff map'  units='mult'  use_header_enum=off  row_header_enum={}  col_header_enum={}  use_min_max=on  min_val=0  max_val=2  use_precision=off  precision=''  gain=1  offset=0  exp=1  use_mototune_group=on  mototune_group=lookup_group(gcb)
  motohawk_calibration2 : MotoHawk_lib/Calibration & Probing Blocks/motohawk_calibration  nam='VEAdaptGain'  val=1  storage=Calibration  show_more=on  name_source=Use Parameter  data_type=Inherit from 'Default Value'  read_level=1  write_level=1  ovr_cals=on  view_as=Number  enum_struct={'Disabled', 'Enabled'}  vector_style=Wide Row  use_help_units=on  help="'Gain for updating VE table.  This fraction of the error is added to the map every 5ms.'"  units=''  use_header_enum=off  row_header_enum={}  col_header_enum={}  use_min_max=on  min_val=0  max_val=1  use_precision=off  precision='8.6'  gain=1  offset=0  exp=1  use_mototune_group=on  mototune_group=lookup_group(gcb)
  motohawk_probe1 : MotoHawk_lib/Calibration & Probing Blocks/motohawk_probe  nam='VolEff_Error'  show_more=on  name_source=Use Parameter  read_level=1  view_as=Number  enum_struct={'Disabled', 'Enabled'}  vector_style=Wide Row  use_help_units=on  help='Error in Volumetric Efficiency at the current operating point, as compared to MAF sensor'  units=''  use_header_enum=off  row_header_enum={}  col_header_enum={}  use_precision=off  precision=''  gain=1  offset=0  exp=1  use_mototune_group=on  mototune_group=lookup_group(gcb)
  motohawk_probe2 : MotoHawk_lib/Calibration & Probing Blocks/motohawk_probe  nam='MAF_ModelError'  show_more=on  name_source=Use Parameter  read_level=1  view_as=Number  enum_struct={'Disabled', 'Enabled'}  vector_style=Wide Row  use_help_units=on  help='Air Mass Flow Rate error, as compared to MAF sensor'  units='g/s'  use_header_enum=off  row_header_enum={}  col_header_enum={}  use_precision=off  precision=''  gain=1  offset=0  exp=1  use_mototune_group=on  mototune_group=lookup_group(gcb)
  motohawk_probe3 : MotoHawk_lib/Calibration & Probing Blocks/motohawk_probe  nam='VEAdapting'  show_more=on  name_source=Use Parameter  read_level=1  view_as=Enumeration  enum_struct={'Not adapting', 'Adapting'}  vector_style=Wide Row  use_help_units=on  help='Indicates whether the volumetric efficiency map is currently being adjusted'  units=''  use_header_enum=off  row_header_enum={}  col_header_enum={}  use_precision=off  precision=''  gain=1  offset=0  exp=1  use_mototune_group=on  mototune_group=lookup_group(gcb)
  wires:
  Product0/1 -> Adapt VolEff Map/1(Error)
  motohawk_calibration2/1 -> Product0/2
  MAF_Model [g/s]/1 -> Safe Divide/2(Inport), Sum1/2
  MAF_Sensor [g/s]/1 -> Sum1/1
  Sum1/1 -> Safe Divide/1(X), motohawk_probe2/1
  Safe Divide/1(" ") -> Abs/1, motohawk_probe1/1, Product0/1
  motohawk_calibration1/1 -> Relational Operator/2
  Relational Operator/1 -> Logical Operator/3
  Abs/1 -> Relational Operator/1
  SSEngOpr [bool]/1 -> Logical Operator/2
  Logical Operator/1 -> motohawk_probe3/1, Adapt VolEff Map/Enable, Adapt VolEff Map/2(AdaptEnabled)
  motohawk_calibration/1 -> Logical Operator/1
  VE/1 -> Adapt VolEff Map/3(VE)

== system motohawk_engine_motoshare_lib/Speed Density - MAP Referenced - Adaptive/C to K1 ==
  C : Inport
  C to K : Fcn  Expr=u(1) + 273.2
  K : Outport
  wires:
  C to K/1 -> K/1
  C/1 -> C to K/1

== system motohawk_engine_motoshare_lib/Idle Governor/Idle State Determination/Determine if RPM is Falling ==
  note: Determine whether RPM is falling
  RPM : Inport
  Derivitive : motohawk_control_primitives_lib/Derivitive  samp_time=-1
  Falling RPM is Negative Derivative : Gain  Gain=-1
  Median Filter : motohawk_control_primitives_lib/Median Filter  buffer_size=17
  Relational Operator : RelationalOperator  Operator=<
  motohawk_calibration : MotoHawk_lib/Calibration & Probing Blocks/motohawk_calibration  nam='RPMFallingRate'  val=4  storage=Calibration  show_more=on  name_source=Use Parameter  data_type=Inherit from 'Default Value'  read_level=1  write_level=1  ovr_cals=on  view_as=Number  enum_struct={'Disabled', 'Enabled'}  vector_style=Wide Row  use_help_units=on  help='The minimum rate of change in RPM that triggers RPMFalling - This should be a positive value'  units='RPM/sec'  use_header_enum=off  row_header_enum={}  col_header_enum={}  use_min_max=on  min_val=0  max_val=1000  use_precision=off  precision=''  gain=1  offset=0  exp=1  use_mototune_group=off  mototune_group=motohawk_vardec_path(gcb)
  motohawk_probe : MotoHawk_lib/Calibration & Probing Blocks/motohawk_probe  nam='RPMFalling'  show_more=off  name_source=Use Parameter  read_level=1  view_as=Number  enum_struct={'Disabled', 'Enabled'}  vector_style=Wide Row  use_help_units=off  help=''  units=''  use_header_enum=off  row_header_enum={}  col_header_enum={}  use_precision=off  precision=''  gain=1  offset=0  exp=1  use_mototune_group=off  mototune_group=motohawk_vardec_path(gcb)
  RPM Falling : Outport
  wires:
  Falling RPM is Negative Derivative/1 -> Relational Operator/2
  RPM/1 -> Derivitive/1
  Relational Operator/1 -> RPM Falling/1, motohawk_probe/1
  motohawk_calibration/1 -> Falling RPM is Negative Derivative/1
  Median Filter/1 -> Relational Operator/1
  Derivitive/1 -> Median Filter/1
